simulink model "boost_openloop_branch_b"  (R2026a)
settings: Solver=ode1  StopTime=0.04  FixedStep=5e-07
PreLoadFcn:
  | load('/Users/arkadiyturevskiy/Documents/Claude/ACtive Learning/active_learning_rom/tests/models/boost_openloop_branch_b_data.mat');
values from neighbouring files (symbols this model uses):
  lut_delta_iL = [0.0625 0.125 0.1875 0.25 0.3125 0.375 0.4375 0.5 0.5625 0.625 0.6875 0.75 ... (17 elements, 1x17)]    [boost_openloop_branch_b_data.mat]
  lut_duty = [0.05 0.1 0.15 0.2 0.25 0.3 0.35 0.4 0.45 0.5 0.55 0.6 ... (17 elements, 1x17)]    [boost_openloop_branch_b_data.mat]
  rom_A_iL = [0.999687614159 -124.83363368 4.98578472344e-06 0.994215151695 0.999762668551 -94.8622569536 4.9890945696e-06 0.995561889449 0.999774545291 -90.1161803197 4.98926742974e-06 0.995634892728 ... (48 elements, 2x2x12)]    [boost_openloop_branch_b_data.mat]
  rom_A_vout = [0.997679826063 0.0224896776117 -0.0224896776117 0.996844301515 0.99813562051 0.0215642924489 -0.0215642924489 0.997211281317 0.997886719753 0.0201644867418 -0.0201644867418 0.997746081585 ... (48 elements, 2x2x12)]    [boost_openloop_branch_b_data.mat]
  rom_B_iL = [1.24765138145e-11 4.98578472344e-06 1.24819826275e-11 4.9890945696e-06 1.24822626786e-11 4.98926742974e-06 1.2486087123e-11 4.99157296543e-06 1.24852789471e-11 4.99109170393e-06 1.24673861306e-11 4.98038494046e-06 ... (24 elements, 2x1x12)]    [boost_openloop_branch_b_data.mat]
  rom_B_vout = [-0.000659605146775 0.000685474392838 -0.000633677458221 0.000705978748011 -0.000738709016608 0.000680131849291 -0.000780919952946 0.000632973710817 -0.000781580752914 0.000733691582428 -0.000623926175584 0.00102911630671 ... (24 elements, 2x1x12)]    [boost_openloop_branch_b_data.mat]
  rom_C_iL = [81080609.5466 351727.785265 72058385.1195 463245.102909 80793898.1348 428314.698057 84783313.3576 412202.772785 100311106.162 339038.977163 94505422.5177 738979.532814 ... (24 elements, 1x2x12)]    [boost_openloop_branch_b_data.mat]
  rom_C_vout = [-130.505079393 -138.776877641 -125.307272762 -142.741402093 -146.502843497 -137.654984472 -155.097411519 -128.183600825 -155.126692814 -148.244405015 -122.994669777 -207.674997227 ... (24 elements, 1x2x12)]    [boost_openloop_branch_b_data.mat]
  rom_grid = [0.15 0.2 0.25 0.3 0.35 0.4 0.45 0.5 0.55 0.6 0.65 0.7]    [boost_openloop_branch_b_data.mat]
  rom_iL_ss = [0.98814697912 1.12510002478 1.29195775539 1.49760168395 1.75446144619 2.08035874156 2.50157277977 3.05814667259 3.81227502452 4.8671289089 6.40662786902 8.77935103378]    [boost_openloop_branch_b_data.mat]
  rom_state_ic_iL = [0 0 0.15]    [boost_openloop_branch_b_data.mat]
  rom_state_ic_vout = [0 0 0.15]    [boost_openloop_branch_b_data.mat]
  rom_Ts = 5e-06    [boost_openloop_branch_b_data.mat]
  rom_Vout_ss = [5.07777166876 5.44408285414 5.8590553751 6.33306809407 6.87967477571 7.51691754113 8.26935045707 9.17126493353 10.272591593 11.6468742876 13.4096525674 15.7521254903]    [boost_openloop_branch_b_data.mat]
settings Model: Creator=arkadiyturevskiy  LastModifiedBy=arkadiyturevskiy

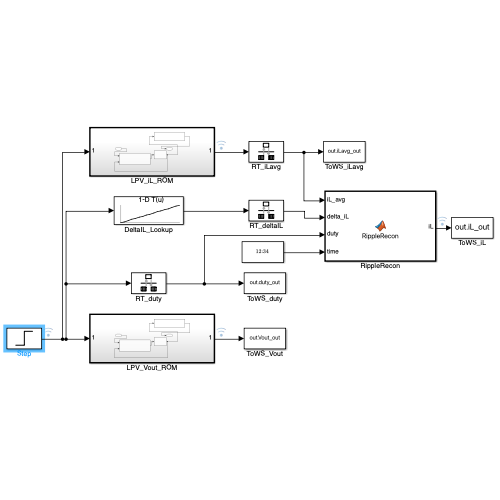
[thumbnail: Simulink's stored preview of the top-level diagram]
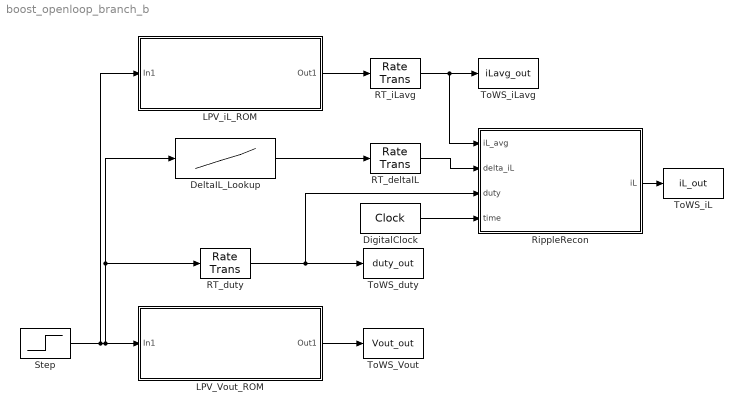
== system boost_openloop_branch_b ==
  DeltaIL_Lookup : Lookup_n-D  NumberOfTableDimensions=1  BreakpointsForDimension1=lut_duty  Table=lut_delta_iL  ExtrapMethod=Clip  InternalRulePriority=Speed  RndMeth=Simplest
  DigitalClock : DigitalClock  SampleTime=5e-07
  LPV_Vout_ROM : Subsystem  TreatAsAtomicUnit=on  SystemSampleTime=5e-06
      settings: MinAlgLoopOccurrences=on
  LPV_iL_ROM : Subsystem  TreatAsAtomicUnit=on  SystemSampleTime=5e-06
      settings: MinAlgLoopOccurrences=on
  RT_deltaIL : RateTransition  OutPortSampleTime=5e-07
  RT_duty : RateTransition  OutPortSampleTime=5e-07
  RT_iLavg : RateTransition  OutPortSampleTime=5e-07
  RippleRecon : MATLAB Function  TreatAsAtomicUnit=on
  Step : Step  Time=0.02  InitialValue=0.3  FinalValue=0.6  SampleTime=0
  ToWS_Vout : ToWorkspace  VariableName=Vout_out  SaveFormat=Timeseries  SampleTime=5e-06
  ToWS_duty : ToWorkspace  VariableName=duty_out  SaveFormat=Timeseries  SampleTime=5e-06
  ToWS_iL : ToWorkspace  VariableName=iL_out  SaveFormat=Timeseries  SampleTime=5e-07
  ToWS_iLavg : ToWorkspace  VariableName=iLavg_out  SaveFormat=Timeseries  SampleTime=5e-06
  wires:
  RT_iLavg/1 -> ToWS_iLavg/1, RippleRecon/1(iL_avg)
  RT_duty/1 -> ToWS_duty/1, RippleRecon/3(duty)
  RippleRecon/1(iL) -> ToWS_iL/1
  LPV_Vout_ROM/1(Out1) -> ToWS_Vout/1
  DeltaIL_Lookup/1 -> RT_deltaIL/1
  DigitalClock/1 -> RippleRecon/4(time)
  RT_deltaIL/1 -> RippleRecon/2(delta_iL)
  LPV_iL_ROM/1(Out1) -> RT_iLavg/1
  Step/1 -> DeltaIL_Lookup/1, RT_duty/1, LPV_Vout_ROM/1(In1), LPV_iL_ROM/1(In1)

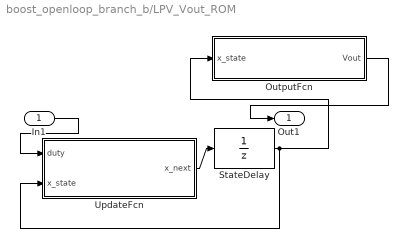
== system boost_openloop_branch_b/LPV_Vout_ROM ==
  In1 : Inport
  OutputFcn : MATLAB Function  TreatAsAtomicUnit=on
  StateDelay : UnitDelay  InitialCondition=rom_state_ic_vout  SampleTime=5e-06
  UpdateFcn : MATLAB Function  TreatAsAtomicUnit=on
  Out1 : Outport
  wires:
  In1/1 -> UpdateFcn/1(duty)
  StateDelay/1 -> OutputFcn/1(x_state), UpdateFcn/2(x_state)
  UpdateFcn/1(x_next) -> StateDelay/1
  OutputFcn/1(Vout) -> Out1/1

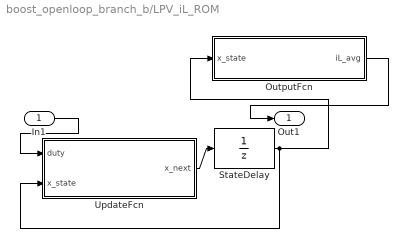
== system boost_openloop_branch_b/LPV_iL_ROM ==
  In1 : Inport
  OutputFcn : MATLAB Function  TreatAsAtomicUnit=on
  StateDelay : UnitDelay  InitialCondition=rom_state_ic_iL  SampleTime=5e-06
  UpdateFcn : MATLAB Function  TreatAsAtomicUnit=on
  Out1 : Outport
  wires:
  In1/1 -> UpdateFcn/1(duty)
  StateDelay/1 -> OutputFcn/1(x_state), UpdateFcn/2(x_state)
  UpdateFcn/1(x_next) -> StateDelay/1
  OutputFcn/1(iL_avg) -> Out1/1

== matlab function boost_openloop_branch_b/LPV_Vout_ROM/UpdateFcn ==
  data: duty input; x_next output; x_state input; rom_A_vout parameter; rom_B_vout parameter; rom_grid parameter; rom_Ts parameter
function x_next = UpdateFcn(duty, x_state, rom_A_vout, rom_B_vout, rom_grid, rom_Ts)
%#codegen
% LPV state update with slowly-tracking reference filter.

nx = size(rom_A_vout, 1);
n_pts = size(rom_A_vout, 3);

x_lpv = x_state(1:nx);
p_ref = x_state(nx+1);

% Clamp duty to grid range
duty_c = max(rom_grid(1), min(rom_grid(n_pts), duty));

% Slowly-tracking reference filter (tau = 0.5ms)
tau_ref = 50e-6;  % Fast tracking (1 switching period) — minimal phase lag
alpha_ref = rom_Ts / (tau_ref + rom_Ts);
p_new = (1 - alpha_ref) * p_ref + alpha_ref * duty_c;
p_new = max(rom_grid(1), min(rom_grid(n_pts), p_new));

% Find interpolation index (codegen-compatible loop)
idx = 1;
for k = 1:n_pts
    if rom_grid(k) <= p_new
        idx = k;
    end
end
if idx >= n_pts
    idx = n_pts - 1;
end
alph = (p_new - rom_grid(idx)) / (rom_grid(idx+1) - rom_grid(idx));

A_k = (1 - alph) * rom_A_vout(:,:,idx) + alph * rom_A_vout(:,:,idx+1);
B_k = (1 - alph) * rom_B_vout(:,:,idx) + alph * rom_B_vout(:,:,idx+1);

% Perturbation input
du = duty_c - p_new;
x_lpv_new = A_k * x_lpv + B_k * du;

% Pack next state
x_next = [x_lpv_new; p_new];

== matlab function boost_openloop_branch_b/LPV_Vout_ROM/OutputFcn ==
  data: x_state input; Vout output; rom_A_vout parameter; rom_C_vout parameter; rom_grid parameter; rom_Vout_ss parameter
function Vout = OutputFcn(x_state, rom_A_vout, rom_C_vout, rom_grid, rom_Vout_ss)
%#codegen
% Compute Vout from LPV state. No duty input -> no direct feedthrough.

nx = size(rom_A_vout, 1);
n_pts = size(rom_A_vout, 3);

x_lpv = x_state(1:nx);
p_ref = x_state(nx+1);

% Clamp p_ref to grid range
p_c = max(rom_grid(1), min(rom_grid(n_pts), p_ref));

% Find interpolation index (codegen-compatible loop)
idx = 1;
for k = 1:n_pts
    if rom_grid(k) <= p_c
        idx = k;
    end
end
if idx >= n_pts
    idx = n_pts - 1;
end

alph = (p_c - rom_grid(idx)) / (rom_grid(idx+1) - rom_grid(idx));
C_k = (1 - alph) * rom_C_vout(:,:,idx) + alph * rom_C_vout(:,:,idx+1);
y_base = (1 - alph) * rom_Vout_ss(idx) + alph * rom_Vout_ss(idx+1);
Vout = y_base + C_k * x_lpv;

== matlab function boost_openloop_branch_b/LPV_iL_ROM/OutputFcn ==
  data: x_state input; iL_avg output; rom_A_iL parameter; rom_C_iL parameter; rom_grid parameter; rom_iL_ss parameter
function iL_avg = OutputFcn(x_state, rom_A_iL, rom_C_iL, rom_grid, rom_iL_ss)
%#codegen
% Compute iL_avg from LPV state. No duty input -> no direct feedthrough.

nx = size(rom_A_iL, 1);
n_pts = size(rom_A_iL, 3);

x_lpv = x_state(1:nx);
p_ref = x_state(nx+1);

% Clamp p_ref to grid range
p_c = max(rom_grid(1), min(rom_grid(n_pts), p_ref));

% Find interpolation index (codegen-compatible loop)
idx = 1;
for k = 1:n_pts
    if rom_grid(k) <= p_c
        idx = k;
    end
end
if idx >= n_pts
    idx = n_pts - 1;
end

alph = (p_c - rom_grid(idx)) / (rom_grid(idx+1) - rom_grid(idx));
C_k = (1 - alph) * rom_C_iL(:,:,idx) + alph * rom_C_iL(:,:,idx+1);
y_base = (1 - alph) * rom_iL_ss(idx) + alph * rom_iL_ss(idx+1);
iL_avg = y_base + C_k * x_lpv;

== matlab function boost_openloop_branch_b/LPV_iL_ROM/UpdateFcn ==
  data: duty input; x_next output; x_state input; rom_A_iL parameter; rom_B_iL parameter; rom_grid parameter; rom_Ts parameter
function x_next = UpdateFcn(duty, x_state, rom_A_iL, rom_B_iL, rom_grid, rom_Ts)
%#codegen
% LPV state update with slowly-tracking reference filter.

nx = size(rom_A_iL, 1);
n_pts = size(rom_A_iL, 3);

x_lpv = x_state(1:nx);
p_ref = x_state(nx+1);

% Clamp duty to grid range
duty_c = max(rom_grid(1), min(rom_grid(n_pts), duty));

% Slowly-tracking reference filter (tau = 0.5ms)
tau_ref = 50e-6;  % Fast tracking (1 switching period) — minimal phase lag
alpha_ref = rom_Ts / (tau_ref + rom_Ts);
p_new = (1 - alpha_ref) * p_ref + alpha_ref * duty_c;
p_new = max(rom_grid(1), min(rom_grid(n_pts), p_new));

% Find interpolation index (codegen-compatible loop)
idx = 1;
for k = 1:n_pts
    if rom_grid(k) <= p_new
        idx = k;
    end
end
if idx >= n_pts
    idx = n_pts - 1;
end
alph = (p_new - rom_grid(idx)) / (rom_grid(idx+1) - rom_grid(idx));

A_k = (1 - alph) * rom_A_iL(:,:,idx) + alph * rom_A_iL(:,:,idx+1);
B_k = (1 - alph) * rom_B_iL(:,:,idx) + alph * rom_B_iL(:,:,idx+1);

% Perturbation input
du = duty_c - p_new;
x_lpv_new = A_k * x_lpv + B_k * du;

% Pack next state
x_next = [x_lpv_new; p_new];

== matlab function boost_openloop_branch_b/RippleRecon ==
  data: iL_avg input; iL output; delta_iL input; duty input; time input
function iL = RippleRecon(iL_avg, delta_iL, duty, time)
%#codegen
% Reconstruct triangular iL waveform from average and ripple amplitude.
% Runs at 0.5us to capture switching ripple within each 5us PWM period.

Ts_pwm = 5e-6;

% Phase within current PWM period [0, 1)
phase = mod(time, Ts_pwm) / Ts_pwm;

% Clamp duty to avoid division by zero
duty_c = max(0.01, min(0.99, duty));

if phase < duty_c
    % Rising portion: current ramps up during on-time
    iL = iL_avg - delta_iL/2 + delta_iL * (phase / duty_c);
else
    % Falling portion: current ramps down during off-time
    iL = iL_avg + delta_iL/2 - delta_iL * ((phase - duty_c) / (1 - duty_c + eps));
end
